simulink model "CommandBSim"  (R2018b)
settings: Solver=VariableStepAuto  StartTime=0.0  StopTime=10  RelTol=1e-3
libraries: cstblocks x8
settings Model: Creator=olavoie  LastModifiedBy=olavoie

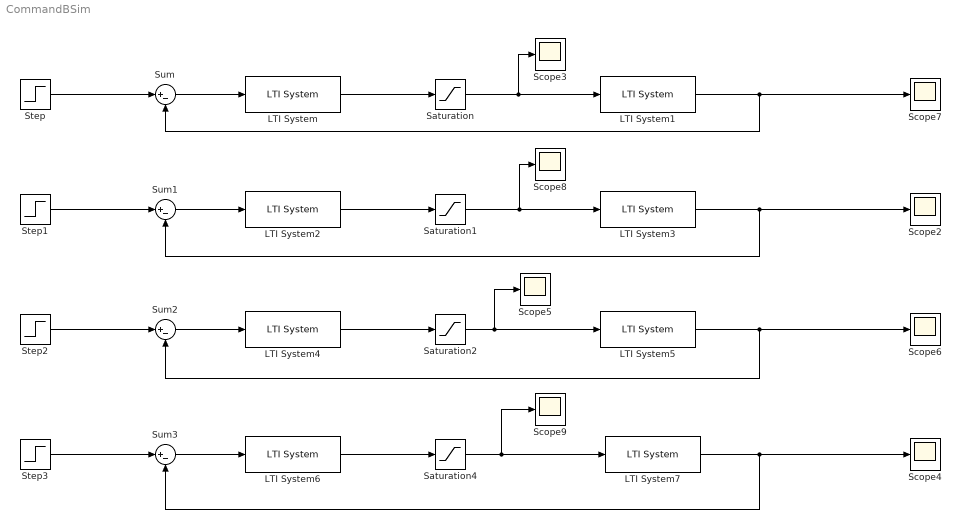
== system CommandBSim ==
  LTI System : cstblocks/LTI System  sys=Cx  IC=[]
  LTI System1 : cstblocks/LTI System  sys=Px  IC=[]
  LTI System2 : cstblocks/LTI System  sys=Cy  IC=[]
  LTI System3 : cstblocks/LTI System  sys=Py  IC=[]
  LTI System4 : cstblocks/LTI System  sys=Cz  IC=[]
  LTI System5 : cstblocks/LTI System  sys=Pz  IC=[]
  LTI System6 : cstblocks/LTI System  sys=Cyaw  IC=[]
  LTI System7 : cstblocks/LTI System  sys=Pyaw  IC=[]
  Saturation{,1..2,4} (4 alike) : Saturate  UpperLimit=110  LowerLimit=-110
  Scope{2..9} (8 alike) : Scope
  Step : Step  Time=0  After=0.5  SampleTime=0  VectorParams1D=off
  Step1 : Step  Time=0  After=0.5  SampleTime=0  VectorParams1D=off
  Step2 : Step  Time=0  After=0.35  SampleTime=0  VectorParams1D=off
  Step3 : Step  Time=0  After=0.5  SampleTime=0  VectorParams1D=off
  Sum{,1..3} (4 alike) : Sum  Inputs=|+-
  wires:
  Sum/1 -> LTI System/1
  LTI System/1 -> Saturation/1
  LTI System3/1 -> Scope2/1, Sum1/2
  Saturation1/1 -> Scope8/1, LTI System3/1
  LTI System2/1 -> Saturation1/1
  Sum1/1 -> LTI System2/1
  LTI System5/1 -> Scope6/1, Sum2/2
  Sum3/1 -> LTI System6/1
  LTI System7/1 -> Scope4/1, Sum3/2
  LTI System6/1 -> Saturation4/1
  Sum2/1 -> LTI System4/1
  Step/1 -> Sum/1
  Step1/1 -> Sum1/1
  Step2/1 -> Sum2/1
  Step3/1 -> Sum3/1
  LTI System4/1 -> Saturation2/1
  Saturation2/1 -> Scope5/1, LTI System5/1
  Saturation/1 -> Scope3/1, LTI System1/1
  Saturation4/1 -> Scope9/1, LTI System7/1
  LTI System1/1 -> Sum/2, Scope7/1
